simulink model "Validacion"  (R2019b)
settings: Solver=ode4  StartTime=0.0  StopTime=10.0  FixedStep=0.01  RelTol=1e-3
libraries: simulink x1
settings Model: Creator=Usuario  LastModifiedBy=Usuario

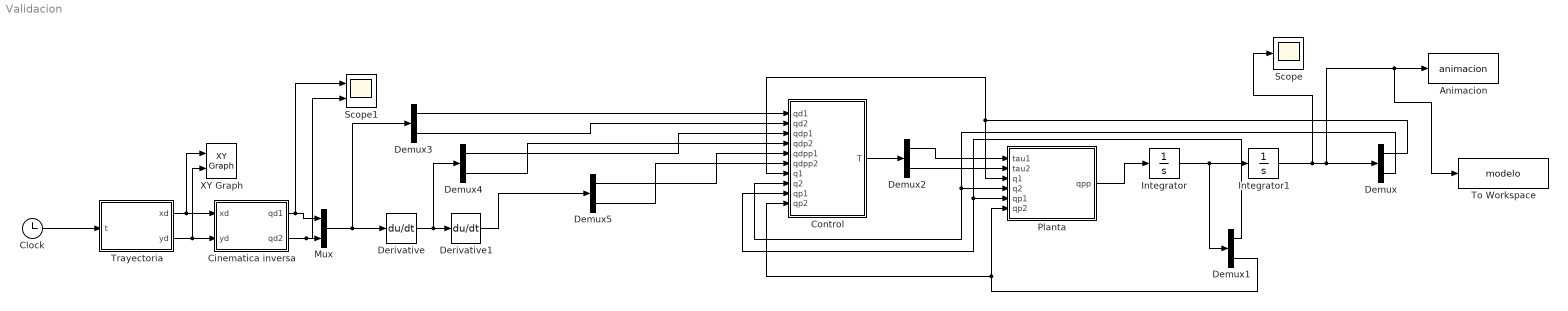
== system Validacion ==
  Animacion : MATLABFcn  MATLABFcn=animacion  OutputDimensions=0
  Cinematica inversa : MATLAB Function  TreatAsAtomicUnit=on
  Clock : Clock
  Control : MATLAB Function  TreatAsAtomicUnit=on
  Demux{,1..5} (6 alike) : Demux  Outputs=2
  Derivative : Derivative
  Derivative1 : Derivative
  Integrator : Integrator
  Integrator1 : Integrator  InitialCondition=[2.71 -1.74]
  Mux : Mux  Inputs=2
  Planta : MATLAB Function  TreatAsAtomicUnit=on
  Scope : Scope
  Scope1 : Scope  NumInputPorts=2
  To Workspace : ToWorkspace  VariableName=modelo  SaveFormat=Timeseries  SampleTime=-1
  Trayectoria : MATLAB Function  TreatAsAtomicUnit=on
  XY Graph : simulink/Sinks/XY Graph  xmin=-1  xmax=1  ymin=-1  ymax=1  st=-1
  wires:
  Planta/1(qpp) -> Integrator/1
  Integrator/1 -> Demux1/1, Integrator1/1
  Integrator1/1 -> Scope/1, To Workspace/1, Animacion/1, Demux/1
  Demux/1 -> Planta/3(q1), Control/7(q1)
  Demux/2 -> Control/8(q2), Planta/4(q2)
  Demux1/1 -> Control/9(qp1), Planta/5(qp1)
  Demux1/2 -> Control/10(qp2), Planta/6(qp2)
  Control/1(T) -> Demux2/1
  Clock/1 -> Trayectoria/1(t)
  Cinematica inversa/1(qd1) -> Scope1/1, Mux/1
  Mux/1 -> Demux3/1, Derivative/1
  Derivative/1 -> Demux4/1, Derivative1/1
  Demux3/1 -> Control/1(qd1)
  Derivative1/1 -> Demux5/1
  Demux3/2 -> Control/2(qd2)
  Demux4/1 -> Control/3(qdp1)
  Demux4/2 -> Control/4(qdp2)
  Demux5/1 -> Control/5(qdpp1)
  Demux5/2 -> Control/6(qdpp2)
  Trayectoria/1(xd) -> XY Graph/1, Cinematica inversa/1(xd)
  Trayectoria/2(yd) -> XY Graph/2, Cinematica inversa/2(yd)
  Demux2/1 -> Planta/1(tau1)
  Demux2/2 -> Planta/2(tau2)
  Cinematica inversa/2(qd2) -> Scope1/2, Mux/2

== matlab function Validacion/Control ==
  data: qd1 input; qd2 input; qdp1 input; qdp2 input; qdpp1 input; qdpp2 input; q1 input; T output; q2 input; qp1 input; qp2 input
function T = fcn(qd1,qd2,qdp1,qdp2,qdpp1,qdpp2,q1,q2,qp1,qp2)
% %%Parametros
% m1=1;l1=1;lc1=0.5;I1=0.01;b1=0.17;
% m2=1;l2=1;lc2=0.5;I2=0.01;b2=0.13;
% g=9.81;
% kp1=15;kp2=10;
% kd1=10;kd2=6;
% %%Ganancias
% Kp11=kp1;
% Kp12=0;
% Kp21=0;
% Kp22=kp2;
% Kp=[Kp11 Kp12;Kp21 Kp22];
% 
% Kd11=kd1;
% Kd12=0;
% Kd21=0;
% Kd22=kp2;
% Kd=[Kd11 Kd12;Kd21 Kd22];
% %%Vector de posicion
% qd1=pi;qd2=0;
% 
% qh=[qd1-q1;qd2-q2];
% qp=[qp1;qp2];
% %%Vector de gravedad
% G1=(m1*lc1+m2*l1)*g*sin(q1)+m2*g*lc2*sin(q1+q2);
% G2=m2*g*lc2*sin(q1+q2);
% G=[G1;G2];
% 
% %%Control P con retro de velocidad mas compesacion de gravedad
% T= Kp*qh-Kd*qp+G;

%%Parametros
m1=0.43453;
l1=141.8/1e3;
lc1=39.164/1e3;
I1=0.00105681;
b1=0.04;
m2= 0.83963;
l2=230.49/1e3;
lc2=80.93/1e3;
I2=0.00481309;
b2=0.002;
g=9.81;
%%Matriz de masas
M11=m1*lc1^2+m2*l1^2+m2*lc2^2+2*m2*l1*lc2*cos(q2)+I1+I2;
M12=m2*lc2^2+m2*l1*lc2*cos(q2)+I2;
M21=m2*lc2^2+m2*l1*lc2*cos(q2)+I2;
M22=m2*lc2^2+I2;
M=[M11 M12;M21 M22];
%%Matriz de inercia
C11=-2*m2*l1*lc2*sin(q2)*qp2;
C12=-m2*l1*lc2*sin(q2)*qp2;
C21=m2*l1*lc2*sin(q2)*qp1;
C22=0;
C = [C11 C12;C21 C22];
%%Matriz diagonal de friccion viscoza
B11=b1;
B12=0;
B21=0;
B22=b2;
B=[B11 B12;B21 B22];
%%Vector de gravedad
G1=(m1*lc1+m2*l1)*g*sin(q1)+m2*g*lc2*sin(q1+q2);
G2=m2*g*lc2*sin(q1+q2);
G=[G1;G2];

kp1=20;kp2=15;
kd1=12;kd2=10;
%%Ganancias
Kp11=kp1;
Kp12=0;
Kp21=0;
Kp22=kp2;
Kp=[Kp11 Kp12;Kp21 Kp22];

Kd11=kd1;
Kd12=0;
Kd21=0;
Kd22=kd2;
Kd=[Kd11 Kd12;Kd21 Kd22];
%%Vector de error posicion
qh=[qd1-q1;qd2-q2];
%%Vector de velocidad
qp=[qp1;qp2];
%%Vector de aceleracion deseada
qdpp=[qdpp1;qdpp2];
%%Vector del error de velocidad
qhp=[qdp1-qp1;qdp2-qp2];
%%Control de par calculado
T=M*(qdpp+Kd*qhp+Kp*qh)+C*qp+B*qp+G;

== matlab function Validacion/Planta ==
  data: tau1 input; tau2 input; q1 input; qpp output; q2 input; qp1 input; qp2 input
function qpp = fcn(tau1,tau2,q1,q2,qp1,qp2)
%%Parametros
m1=0.43453;
l1=141.8/1e3;
lc1=39.164/1e3;
I1=0.00105681;
b1=0.04;
m2= 0.83963;
l2=230.49/1e3;
lc2=80.93/1e3;
I2=0.00481309;
b2=0.002;
g=9.81;
%%Matriz de masas
M11=m1*lc1^2+m2*l1^2+m2*lc2^2+2*m2*l1*lc2*cos(q2)+I1+I2;
M12=m2*lc2^2+m2*l1*lc2*cos(q2)+I2;
M21=m2*lc2^2+m2*l1*lc2*cos(q2)+I2;
M22=m2*lc2^2+I2;
M=[M11 M12;M21 M22];
%%Matriz de inercia
C11=-2*m2*l1*lc2*sin(q2)*qp2;
C12=-m2*l1*lc2*sin(q2)*qp2;
C21=m2*l1*lc2*sin(q2)*qp1;
C22=0;
C = [C11 C12;C21 C22];
%%Matriz diagonal de friccion viscoza
B11=b1;
B12=0;
B21=0;
B22=b2;
B=[B11 B12;B21 B22];
%%Vector de gravedad
G1=(m1*lc1+m2*l1)*g*sin(q1)+m2*g*lc2*sin(q1+q2);
G2=m2*g*lc2*sin(q1+q2);
G=[G1;G2];
%%Vector de posicion
q=[q1;q2];
%%Vector de velocidad
qp=[qp1;qp2];
%%Vector de entrdas
%%tau1=10;tau2=2;
T=[tau1;tau2];
%%Planta
qpp=M\(T-C*qp-B*qp-G);

== matlab function Validacion/Trayectoria ==
  data: t input; xd output; yd output
function [xd,yd] = fcn(t)
%%circulo
hx=0.2;
hy=0;
a=1;
b=2;

T=5;
f=1/T;
w=2*pi*f;
xd=hx+0.05*((a-b)*cos(w*t)+b*cos(w*t*((a/b)-1)));
yd=hy+0.05*((a-b)*sin(w*t)+b*sin(w*t*((a/b)-1)));


% % %lemiscata*
% % a=0.15;
% % hx=0.4;
% % hy=0;
% % T=10;
% % f=1/T;
% % w=2*pi*f;
% % xd=hx+a*cos(w*t)/(1+sin(w*t)^2);
% % yd=hy+a*sin(w*t)*cos(w*t)/(1+sin(w*t)^2);
% %%Flor de 4 petalos
% a=0.02;
% R=0.2;
% n=2;
% hx=0.3;
% hy=0;
% T=10;
% f=1/T;
% w=2*pi*f;
% xd=hx+(a+R*cos(n*w*t)^2)*cos(w*t);
% yd=hy+(a+R*cos(n*w*t)^2)*sin(w*t);

== matlab function Validacion/Cinematica inversa ==
  data: xd input; qd1 output; yd input; qd2 output
function [qd1,qd2] = fcn(xd,yd)

l1=141.8/1e3;l2=230.49/1e3;
cosq2 = (xd^2+yd^2-l1^2-l2^2)/(2*l1*l2);
qd2=atan2(-sqrt(1-cosq2^2),cosq2);
qd1=atan2(xd,-yd)-atan2(l2*sin(qd2),(l1+l2*cos(qd2)));
